simulink model "robot"  (R2022b)
settings: Solver=ode3  StartTime=0.0  StopTime=10.0  FixedStep=0.01  RelTol=1e-3
undefined symbols (not defined in the file or in its folder): DiscIntNeverNeededParam
libraries: simulink x1
settings Model: Creator=Oscar  LastModifiedBy=Oscar

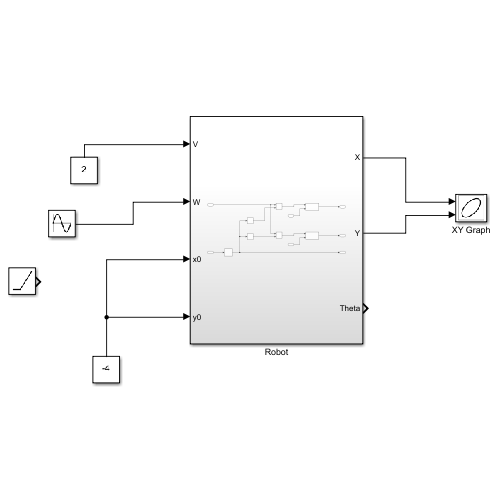
[thumbnail: Simulink's stored preview of the top-level diagram]
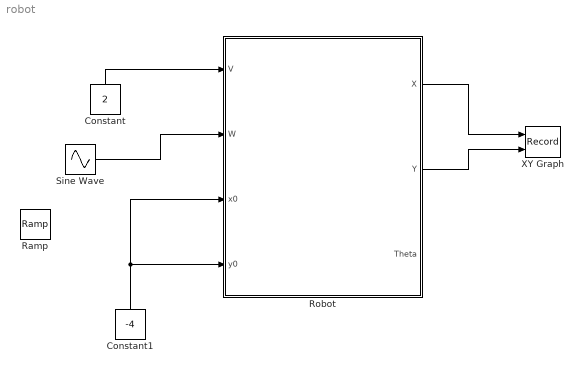
== system robot ==
  Constant : Constant  Value=2
  Constant1 : Constant  Value=-4
  Ramp : simulink/Sources/Ramp  slope=1  start=0  InitialOutput=0
  Robot : Subsystem
  Sine Wave : Sin  Amplitude=10  Frequency=10  SampleTime=0
  XY Graph : Record  FileSettingsInternal="{\"entries\":[{\"content\":{\"excelSettings\":{\"content\":{},\"type\":\"Streamout.ExcelSettings\"}},\"type\":\"Streamout.FileSettingStorage\",\"uuid\":\"1fdc4e21-baea-4552-8ef6-a7e9773fe58a\"}],\"packageUris\":[\"http://schema.mathworks.com/mf0/streamout_blocks/R2020a\"],\"version\":\"1.0\"}"  Layout=[1 1]  SignalsInternal="{\"entries\":[{\"content\":{\"signals\":[{\"content\":{\"blockPath\":[\"robot/XY Graph\"],\"channel\":[],\"dimensions\":[1],\"domain\":\"robot/XY Graph\",\"lineColor\":\"#a2142f\",\"plots\":[1],\"port\":1,\"sid\":[\"\"],\"signalID\":693,\"signalName\":\"Robot:1\"},\"type\":\"RecordBlkView.Signal\",\"uuid\":\"6c2c6d84-a56a-4cfb-ba55-731c135e51ae\"},{\"content\":{\"blockPath\":[\"robot/XY Graph\"],\"channel\":[],\"dimensions\":[1],\"domain\":\"robot/XY Graph\",\"lineColor\":\"#139fff\",\"plots\":[1],\"port\":2,\"sid\":[\"\"],\"signalID\":697,\"signalName\":\"Robot:2\"},\"type\":\"RecordBlkView.Signal\",\"uuid\":\"7cb923d7-3bb5-43c2-bfff-d6117b973872\"}]},\"type\":\"RecordBlkView.InputSignals\",\"uuid\":\"7ac150d0-c38a-4d40-aa80-92fcc8f03e9b\"}],\"packageUris\":[\"http://schema.mathworks.com/mf0/streamout_blocks/R2020a\"],\"version\":\"1.0\"}"  VisualizationBindings="{\"xyplotplugin\":{\"info\":[{\"series\":[{\"bindingParametersList\":[{\"parameter\":\"X-Axis\",\"signalID\":693,\"signalName\":\"Robot:1\"},{\"parameter\":\"Y-Axis\",\"signalID\":697,\"signalName\":\"Robot:2\"}],\"seriesID\":26925}],\"subplotID\":1}]}}"  CompatibilityTag=XY
  wires:
  Constant/1 -> Robot/1(V)
  Robot/1(X) -> XY Graph/1
  Robot/2(Y) -> XY Graph/2
  Sine Wave/1 -> Robot/2(W)
  Constant1/1 -> Robot/4(y0), Robot/3(x0)

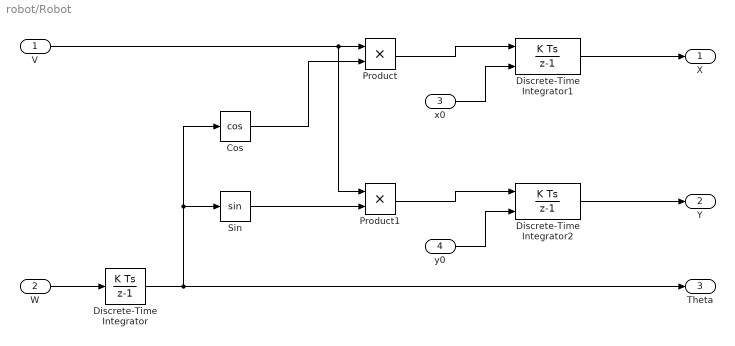
== system robot/Robot ==
  V : Inport
  W : Inport  Port=2
  x0 : Inport  Port=3
  y0 : Inport  Port=4
  Cos : Trigonometry  Operator=cos
  Discrete-Time Integrator : DiscreteIntegrator  SampleTime=-1  ICPrevOutput=DiscIntNeverNeededParam  ICPrevScaledInput=DiscIntNeverNeededParam
  Discrete-Time Integrator1 : DiscreteIntegrator  InitialConditionSource=external  SampleTime=-1  ICPrevOutput=DiscIntNeverNeededParam  ICPrevScaledInput=DiscIntNeverNeededParam
  Discrete-Time Integrator2 : DiscreteIntegrator  InitialConditionSource=external  SampleTime=-1  ICPrevOutput=DiscIntNeverNeededParam  ICPrevScaledInput=DiscIntNeverNeededParam
  Product : Product
  Product1 : Product
  Sin : Trigonometry
  X : Outport
  Y : Outport  Port=2
  Theta : Outport  Port=3
  wires:
  Discrete-Time Integrator/1 -> Theta/1, Sin/1, Cos/1
  Discrete-Time Integrator1/1 -> X/1
  Sin/1 -> Product1/2
  V/1 -> Product1/1, Product/1
  Product1/1 -> Discrete-Time Integrator2/1
  Product/1 -> Discrete-Time Integrator1/1
  Discrete-Time Integrator2/1 -> Y/1
  W/1 -> Discrete-Time Integrator/1
  Cos/1 -> Product/2
  x0/1 -> Discrete-Time Integrator1/2
  y0/1 -> Discrete-Time Integrator2/2
